simulink model "Copy_of_BatteryPack"  (R2023b)
settings: Solver=VariableStepAuto  StartTime=0.0  StopTime=10.0  RelTol=1e-3
InitFcn:
  | eta=0.992943452611046;
  | Q=5.134436834270520;
  | Qinv=1/Q;
  | Qinv_cells=Qinv+0.01*rand(12,1);
  | delta_t=0.1;
  | delta_t_delta=4;
  | taw=2.410723815561624;
  | R0=0.011163238296886;
  | R0_cells=R0+0.001*rand(12,1);
  | R=0.002515135572506;
  | gamma=61.749752200480295;
  | M0=0.002542395121461;
  | M=0.044341699418566;
  | OCV0=[3.03083668947220,3.16996176507765,3.24654613672245,3.30462471088150,3.35178831826018,3.39207985837564,3.42754280925954,3.45930893308633,3.48845834377828,3.51506471884948,3.53941528250350,3.56229005089512,3.58347680139773,3.60345371361795,3.62204667414497,3.63945293994712,3.65555208129593,3.67025842747189,3.68283722926942,3.69256635796299,3.69934356504319,3.70421492193387,3.70864080668278,3.71251647816700,3.71676450243010,3.72076080442289,3.72459036631361,3.72852113964889,3.73262555664002,3.73679788031633,3.74085805813141,3.74504293170943,3.74937151420852,3.75360503345497,3.75808554938499,3.76253512812700,3.76686713224277,3.77129741354356,3.77568299945893,3.78010899552110,3.78432597237866,3.78866667245794,3.79282973590265,3.79699149175738,3.80102646886227,3.80486901671467,3.80859160652083,3.81234290326678,3.81578374146922,3.81901029060391,3.82246264968075,3.82565270541301,3.82878492908885,3.83182846251259,3.83504605065465,3.83817152994830,3.84120926637331,3.84427045104513,3.84745505461551,3.85048527227548,3.85338258086535,3.85633375142700,3.85903736950342,3.86183294078638,3.86426909473005,3.86668409269911,3.86884960464201,3.87075062579497,3.87260151166861,3.87419873493045,3.87590354579771,3.87742660309802,3.87888623494178,3.88013778482297,3.88172955555187,3.88298517380087,3.88445139467736,3.88588841874555,3.88718906620625,3.88865483707461,3.89034900018679,3.89177308296385,3.89345014882802,3.89492324307466,3.89656804158261,3.89814831273987,3.89970800088682,3.90138268502894,3.90325919869100,3.90466035566401,3.90650715226313,3.90818394205928,3.90991726595604,3.91178869314647,3.91353048350435,3.91535717290223,3.91722943087205,3.91902077537227,3.92094773764149,3.92272669049051,3.92480210727778,3.92665898861166,3.92855163124444,3.93049425931182,3.93233822864100,3.93413808807444,3.93586787406902,3.93781878301823,3.93970352375448,3.94141217835583,3.94337738846496,3.94524781610469,3.94705512196599,3.94889596931986,3.95072813117993,3.95268786149774,3.95437483545637,3.95614043217004,3.95813802002780,3.95988737276266,3.96180145819164,3.96333094922522,3.96513598465409,3.96688905019200,3.96847526303094,3.97032227257873,3.97189764460202,3.97357890138617,3.97507568580842,3.97666308363629,3.97834004990894,3.97972757215233,3.98134719919954,3.98282452838428,3.98434240750033,3.98579080664983,3.98712095624815,3.98848186479248,3.99005169119157,3.99140961007081,3.99272279272243,3.99405266719970,3.99553040552875,3.99686295933407,3.99826042332052,3.99959085613132,4.00118770124588,4.00258756750194,4.00410831223298,4.00564378913664,4.00733579962478,4.00874100440808,4.01049664802522,4.01229894715480,4.01403904622199,4.01578258632489,4.01777261837808,4.01971351876421,4.02181419747090,4.02405411757281,4.02634132187682,4.02844966043338,4.03074821161091,4.03287252710406,4.03519979075052,4.03714724603729,4.03920059502787,4.04119005170582,4.04311251958802,4.04485629277420,4.04687276700581,4.04856655229106,4.05028282064349,4.05188790780758,4.05367115501827,4.05540888556017,4.05715082708000,4.05891707849673,4.06058066558082,4.06255984784218,4.06443355862160,4.06646437679668,4.06828978114252,4.07040446117501,4.07260180541029,4.07472443659757,4.07695226365058,4.07952388568996,4.08211497603818,4.08494517654941,4.08785760361077,4.09108975271414,4.09441257923899,4.09808703497329,4.10213358582538,4.10639223642507,4.11114147862302,4.11656968526475,4.12276605724301,4.13028542232852,4.14480757713318];
  | OCVrel=[-0.000420362949371303,-0.000578339102606499,-0.000548212633161139,-0.000532050376255593,-0.000513855468461292,-0.000495687320522634,-0.000487643250941371,-0.000470920985950642,-0.000461928451583620,-0.000448574992511236,-0.000430345291794665,-0.000415864789930715,-0.000403503275736067,-0.000392608506451838,-0.000381149699535297,-0.000369136346590911,-0.000348156127830507,-0.000324184515919599,-0.000280229092973681,-0.000201932662233446,-0.000110744926726894,-3.79084757376537e-05,7.34820416665105e-08,1.98249344364182e-05,1.89028531032423e-05,1.52778169972465e-05,1.34924868477160e-05,9.23542420261725e-06,-1.46245586440975e-06,-1.45311365618779e-05,-2.47366010229282e-05,-3.53430095058658e-05,-4.35761509840300e-05,-4.95443607046995e-05,-5.59569418266839e-05,-5.71405250985218e-05,-5.58628466608733e-05,-5.23710248925624e-05,-5.22024906444821e-05,-5.10066281299635e-05,-4.60070072284917e-05,-4.39210588487260e-05,-4.17087376582674e-05,-3.79965319780425e-05,-3.52883378328963e-05,-2.96358522826692e-05,-1.93487210265394e-05,-1.76654799578108e-05,-1.10481636980021e-05,-6.29033346947879e-06,-6.43729682754031e-06,-8.99082338466702e-06,-5.97476480532998e-06,-4.62198779734926e-06,-8.45626888598137e-06,-3.55310580626464e-06,1.21105779784145e-06,3.23270957394308e-06,4.65975925632772e-06,6.06047576788568e-06,1.06741421249725e-05,1.27740668978125e-05,1.58322240631086e-05,1.58226143080902e-05,1.77356396535024e-05,1.67297263145319e-05,2.20422014608934e-05,3.24455524629346e-05,4.53671310943400e-05,6.36631547519500e-05,7.65783816690908e-05,9.78737779086299e-05,0.000118072210378981,0.000145052733908454,0.000159053964033644,0.000178615115542580,0.000192951944721033,0.000203745870809340,0.000215887472157157,0.000217389449254637,0.000214080259255523,0.000217368801393146,0.000210680488604522,0.000216791472310507,0.000210807141665482,0.000206892775031066,0.000209889448971827,0.000206480366569060,0.000197477832361696,0.000201878205171392,0.000195991461516702,0.000193299624131949,0.000189225295900371,0.000183015755985024,0.000181030375137689,0.000179058026812520,0.000172630244233569,0.000169739554492468,0.000168470860940041,0.000165673583835095,0.000158761613569570,0.000158310548246597,0.000160768730786868,0.000159274891317150,0.000163654237071923,0.000165646854650985,0.000171009006229332,0.000172960872040281,0.000174059186593325,0.000184792008315373,0.000185457536514424,0.000188497928404933,0.000193540560057086,0.000201967121634793,0.000208651810099923,0.000210203310502306,0.000221327742354831,0.000226934798568295,0.000229022527795167,0.000235980838038274,0.000237393722897026,0.000251416377586933,0.000255669183930939,0.000259582507624291,0.000271756110286130,0.000271428141354407,0.000280338423121521,0.000282159563486788,0.000293698306662556,0.000294690382734668,0.000296368480075595,0.000305852381154249,0.000305547730725772,0.000310124564075650,0.000308910141248888,0.000310910207998593,0.000317136879477080,0.000319966110029179,0.000317781933009713,0.000319714895363342,0.000323633211007860,0.000324670146330631,0.000321258389806546,0.000325090635960723,0.000325756317802870,0.000329299487485483,0.000323022114762843,0.000329687741218402,0.000331335077114761,0.000334366863810491,0.000334190313302610,0.000348244516476559,0.000353619969496185,0.000370645612717080,0.000387424759796793,0.000412712601107454,0.000432980002313212,0.000458081645703528,0.000475316126710853,0.000488710969037302,0.000490229811285922,0.000496997034255361,0.000490732502998424,0.000485413024014050,0.000470031399074122,0.000464225038785084,0.000453594366571016,0.000442947689735187,0.000432361194051228,0.000426870028472560,0.000412534978795853,0.000404144406879032,0.000399500637103100,0.000395361789641937,0.000391903989806764,0.000388094198725783,0.000384493593513828,0.000380890719331740,0.000381944387481867,0.000375725748044827,0.000377689116895975,0.000371263292977880,0.000375401761542324,0.000371961214504098,0.000372140497419301,0.000376623010739057,0.000379713082469440,0.000373305112977953,0.000376271071938692,0.000374048457576144,0.000373866132643822,0.000368451986163444,0.000366513632840686,0.000361449855405437,0.000355758001511034,0.000351852945592445,0.000340424192937049,0.000323803410913197,0.000299570003101876,0.000255297108741397,9.12380218506306e-05];
  | soc_values=[0,0.00500000000000000,0.0100000000000000,0.0150000000000000,0.0200000000000000,0.0250000000000000,0.0300000000000000,0.0350000000000000,0.0400000000000000,0.0450000000000000,0.0500000000000000,0.0550000000000000,0.0600000000000000,0.0650000000000000,0.0700000000000000,0.0750000000000000,0.0800000000000000,0.0850000000000000,0.0900000000000000,0.0950000000000000,0.100000000000000,0.105000000000000,0.110000000000000,0.115000000000000,0.120000000000000,0.125000000000000,0.130000000000000,0.135000000000000,0.140000000000000,0.145000000000000,0.150000000000000,0.155000000000000,0.160000000000000,0.165000000000000,0.170000000000000,0.175000000000000,0.180000000000000,0.185000000000000,0.190000000000000,0.195000000000000,0.200000000000000,0.205000000000000,0.210000000000000,0.215000000000000,0.220000000000000,0.225000000000000,0.230000000000000,0.235000000000000,0.240000000000000,0.245000000000000,0.250000000000000,0.255000000000000,0.260000000000000,0.265000000000000,0.270000000000000,0.275000000000000,0.280000000000000,0.285000000000000,0.290000000000000,0.295000000000000,0.300000000000000,0.305000000000000,0.310000000000000,0.315000000000000,0.320000000000000,0.325000000000000,0.330000000000000,0.335000000000000,0.340000000000000,0.345000000000000,0.350000000000000,0.355000000000000,0.360000000000000,0.365000000000000,0.370000000000000,0.375000000000000,0.380000000000000,0.385000000000000,0.390000000000000,0.395000000000000,0.400000000000000,0.405000000000000,0.410000000000000,0.415000000000000,0.420000000000000,0.425000000000000,0.430000000000000,0.435000000000000,0.440000000000000,0.445000000000000,0.450000000000000,0.455000000000000,0.460000000000000,0.465000000000000,0.470000000000000,0.475000000000000,0.480000000000000,0.485000000000000,0.490000000000000,0.495000000000000,0.500000000000000,0.505000000000000,0.510000000000000,0.515000000000000,0.520000000000000,0.525000000000000,0.530000000000000,0.535000000000000,0.540000000000000,0.545000000000000,0.550000000000000,0.555000000000000,0.560000000000000,0.565000000000000,0.570000000000000,0.575000000000000,0.580000000000000,0.585000000000000,0.590000000000000,0.595000000000000,0.600000000000000,0.605000000000000,0.610000000000000,0.615000000000000,0.620000000000000,0.625000000000000,0.630000000000000,0.635000000000000,0.640000000000000,0.645000000000000,0.650000000000000,0.655000000000000,0.660000000000000,0.665000000000000,0.670000000000000,0.675000000000000,0.680000000000000,0.685000000000000,0.690000000000000,0.695000000000000,0.700000000000000,0.705000000000000,0.710000000000000,0.715000000000000,0.720000000000000,0.725000000000000,0.730000000000000,0.735000000000000,0.740000000000000,0.745000000000000,0.750000000000000,0.755000000000000,0.760000000000000,0.765000000000000,0.770000000000000,0.775000000000000,0.780000000000000,0.785000000000000,0.790000000000000,0.795000000000000,0.800000000000000,0.805000000000000,0.810000000000000,0.815000000000000,0.820000000000000,0.825000000000000,0.830000000000000,0.835000000000000,0.840000000000000,0.845000000000000,0.850000000000000,0.855000000000000,0.860000000000000,0.865000000000000,0.870000000000000,0.875000000000000,0.880000000000000,0.885000000000000,0.890000000000000,0.895000000000000,0.900000000000000,0.905000000000000,0.910000000000000,0.915000000000000,0.920000000000000,0.925000000000000,0.930000000000000,0.935000000000000,0.940000000000000,0.945000000000000,0.950000000000000,0.955000000000000,0.960000000000000,0.965000000000000,0.970000000000000,0.975000000000000,0.980000000000000,0.985000000000000,0.990000000000000,0.995000000000000,1];
  | OCV_values=OCV0+25*OCVrel;
  | dZ = soc_values(2) - soc_values(1); % Find spacing of SOC vector
  | dUdZ = diff(OCV_values)/dZ; % Scaled forward finite difference
  | dOCV = ([dUdZ(1) dUdZ] + [dUdZ dUdZ(end)])/2; % Avg of fwd/bkwd diffs
  | SigmaX0 = diag([1e-3 1e-3 1e-2]); % uncertainty of initial state
  | sigmaV = 2e-1; % uncertainty of voltage sensor, output equation
  | sigmaW = 1e1; % uncertainty of current sensor, state equation
  | vbar=0;
  | w_bar=0;
  | nR=0.004;
  | nQ=0.05;
  | ek=0.01;
  | Vmax=4.2;
  | Vmin=2.7;
  | Imax=2*Q;
  | Standby=0;
  | Charging=1;
  | Discharging=2;
  | load('BattCrntDrvCycle.mat');
undefined symbols (not defined in the file): AUX0_OV, AUX1_OV, AUX2_OV, AUX3_OV, AUX4_OV, CELL_OV, CELL_UV, CellVoltages, Fault, FAULT_SUM, NCHAN, PackCurrentChg, PackCurrentDis, PackVoltage, Temperature
libraries: fl_lib x38, nesl_utility x25, simulink x15, ee_lib x8, eeGeneralControl x7, batt_lib x7, hdlsllib x3
(part 2 of 3)

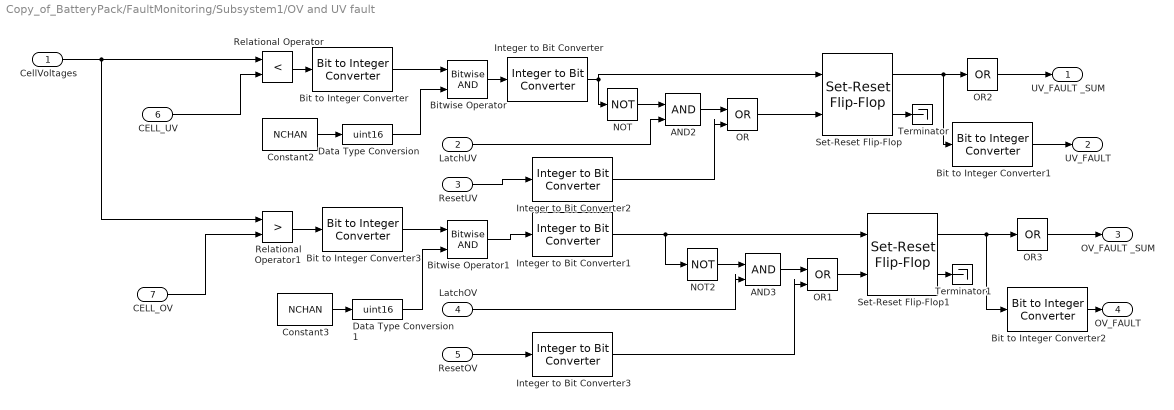
== system Copy_of_BatteryPack/FaultMonitoring/Subsystem1/OV and UV fault ==
  CellVoltages : Inport
  LatchUV : Inport  Port=2
  ResetUV : Inport  Port=3
  LatchOV : Inport  Port=4
  ResetOV : Inport  Port=5
  CELL_UV : Inport  Port=6
  CELL_OV : Inport  Port=7
  AND2 : Logic  IconShape=distinctive  AllPortsSameDT=off  OutDataTypeStr=boolean
  AND3 : Logic  IconShape=distinctive  AllPortsSameDT=off  OutDataTypeStr=boolean
  Bit to Integer Converter{,1..3} (4 alike) : simulink/Logic and Bit Operations/Bit to Integer Converter  nbits=16  bitOrder=MSB first  signedOutputValues=Unsigned  outDtype=Inherit via internal rule  outDtypeSigned=Inherit via internal rule
  Bitwise Operator : simulink/Logic and Bit Operations/Bitwise Operator  logicop=AND  UseBitMask=off  NumInputPorts=2  BitMask=bin2dec('11011001')  BitMaskRealWorld=Stored Integer
  Bitwise Operator1 : simulink/Logic and Bit Operations/Bitwise Operator  logicop=AND  UseBitMask=off  NumInputPorts=2  BitMask=bin2dec('11011001')  BitMaskRealWorld=Stored Integer
  Constant2 : Constant  Value=NCHAN
  Constant3 : Constant  Value=NCHAN
  Data Type Conversion : DataTypeConversion  OutDataTypeStr=uint16  SaturateOnIntegerOverflow=off  RndMeth=Floor
  Data Type Conversion1 : DataTypeConversion  OutDataTypeStr=uint16  SaturateOnIntegerOverflow=off  RndMeth=Floor
  Integer to Bit Converter{,1..3} (4 alike) : simulink/Logic and Bit Operations/Integer to Bit Converter  nbits=16  signedInputValues=Unsigned  bitOrder=MSB first  outDtype=Inherit via internal rule
  NOT : Logic  Operator=NOT  IconShape=distinctive  AllPortsSameDT=off  OutDataTypeStr=boolean
  NOT2 : Logic  Operator=NOT  IconShape=distinctive  AllPortsSameDT=off  OutDataTypeStr=boolean
  OR : Logic  Operator=OR  IconShape=distinctive  AllPortsSameDT=off  OutDataTypeStr=boolean
  OR1 : Logic  Operator=OR  IconShape=distinctive  AllPortsSameDT=off  OutDataTypeStr=boolean
  OR2 : Logic  Operator=OR  Inputs=1  IconShape=distinctive  AllPortsSameDT=off  OutDataTypeStr=boolean
  OR3 : Logic  Operator=OR  Inputs=1  IconShape=distinctive  AllPortsSameDT=off  OutDataTypeStr=boolean
  Relational Operator : RelationalOperator  Operator=<  OutDataTypeStr=boolean  RndMeth=Simplest  InputSameDT=off
  Relational Operator1 : RelationalOperator  Operator=>  OutDataTypeStr=boolean  RndMeth=Simplest  InputSameDT=off
  Set-Reset Flip-Flop : eeGeneralControl/Set-Reset Flip-Flop  LabelModeActiveChoice=Discrete  UndefState=Set  Q0=0  Ts=-1
      settings: LibrarySourceBlock=ee_sl_lib/General Control/Set-Reset Flip-Flop
  Set-Reset Flip-Flop1 : eeGeneralControl/Set-Reset Flip-Flop  LabelModeActiveChoice=Discrete  UndefState=Set  Q0=0  Ts=-1
      settings: LibrarySourceBlock=ee_sl_lib/General Control/Set-Reset Flip-Flop
  Terminator : Terminator
  Terminator1 : Terminator
  UV_FAULT _SUM : Outport
  UV_FAULT : Outport  Port=2
  OV_FAULT _SUM : Outport  Port=3
  OV_FAULT : Outport  Port=4
  wires:
  CellVoltages/1 -> Relational Operator1/1, Relational Operator/1
  CELL_UV/1 -> Relational Operator/2
  CELL_OV/1 -> Relational Operator1/2
  Relational Operator/1 -> Bit to Integer Converter/1
  Constant2/1 -> Data Type Conversion/1
  Relational Operator1/1 -> Bit to Integer Converter3/1
  Constant3/1 -> Data Type Conversion1/1
  Bitwise Operator/1 -> Integer to Bit Converter/1
  NOT/1 -> AND2/1
  LatchUV/1 -> AND2/2
  AND2/1 -> OR/1
  ResetUV/1 -> Integer to Bit Converter2/1
  OR/1 -> Set-Reset Flip-Flop/2
  Set-Reset Flip-Flop/1 -> Bit to Integer Converter1/1, OR2/1
  AND3/1 -> OR1/1
  ResetOV/1 -> Integer to Bit Converter3/1
  LatchOV/1 -> AND3/2
  NOT2/1 -> AND3/1
  OR1/1 -> Set-Reset Flip-Flop1/2
  Bitwise Operator1/1 -> Integer to Bit Converter1/1
  Set-Reset Flip-Flop/2 -> Terminator/1
  Set-Reset Flip-Flop1/2 -> Terminator1/1
  Set-Reset Flip-Flop1/1 -> Bit to Integer Converter2/1, OR3/1
  OR2/1 -> UV_FAULT _SUM/1
  OR3/1 -> OV_FAULT _SUM/1
  Bit to Integer Converter/1 -> Bitwise Operator/1
  Data Type Conversion/1 -> Bitwise Operator/2
  Integer to Bit Converter/1 -> Set-Reset Flip-Flop/1, NOT/1
  Bit to Integer Converter1/1 -> UV_FAULT/1
  Bit to Integer Converter2/1 -> OV_FAULT/1
  Integer to Bit Converter1/1 -> Set-Reset Flip-Flop1/1, NOT2/1
  Bit to Integer Converter3/1 -> Bitwise Operator1/1
  Data Type Conversion1/1 -> Bitwise Operator1/2
  Integer to Bit Converter2/1 -> OR/2
  Integer to Bit Converter3/1 -> OR1/2

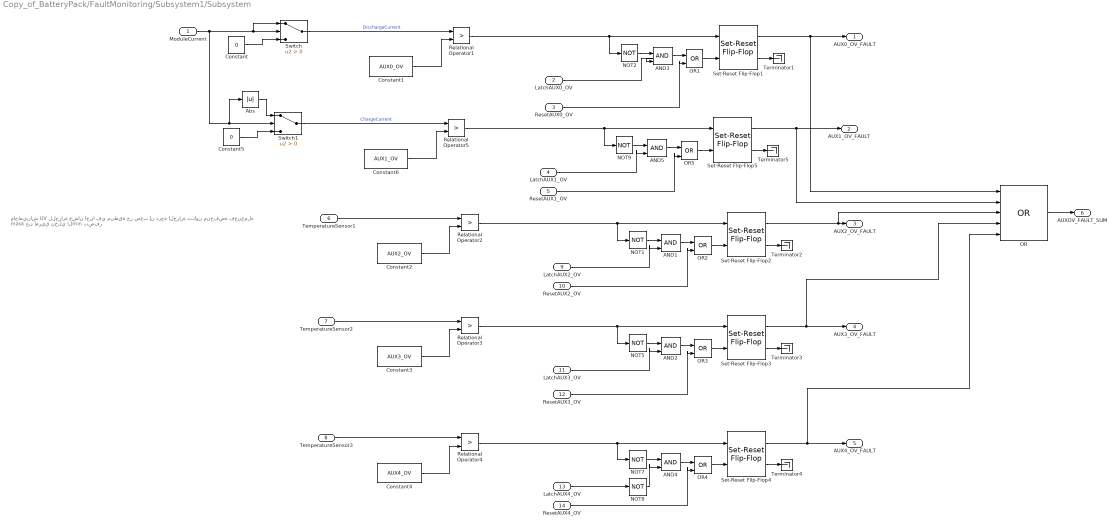
== system Copy_of_BatteryPack/FaultMonitoring/Subsystem1/Subsystem ==
  note: ماحطيناش UV للحرارة عشان احنا في منطقة حر صعب إن درجة الحرارة تكون منخفضة
      | فعنعمله mask عن طريق نخلي الmin بصفر
  ModuleCurrent : Inport
  LatchAUX0_OV : Inport  Port=2
  ResetAUX0_OV : Inport  Port=3
  LatchAUX1_OV : Inport  Port=4
  ResetAUX1_OV : Inport  Port=5
  TemperatureSensor1 : Inport  Port=6
  TemperatureSensor2 : Inport  Port=7
  TemperatureSensor3 : Inport  Port=8
  LatchAUX2_OV : Inport  Port=9
  ResetAUX2_OV : Inport  Port=10
  LatchAUX3_OV : Inport  Port=11
  ResetAUX3_OV : Inport  Port=12
  LatchAUX4_OV : Inport  Port=13
  ResetAUX4_OV : Inport  Port=14
  AND{1..5} (5 alike) : Logic  IconShape=distinctive  AllPortsSameDT=off  OutDataTypeStr=boolean
  Abs : Abs  SaturateOnIntegerOverflow=off
  Constant : Constant  Value=0
  Constant1 : Constant  Value=AUX0_OV
  Constant2 : Constant  Value=AUX2_OV
  Constant3 : Constant  Value=AUX3_OV
  Constant4 : Constant  Value=AUX4_OV
  Constant5 : Constant  Value=0
  Constant6 : Constant  Value=AUX1_OV
  NOT{1..2,5,7..9} (6 alike) : Logic  Operator=NOT  IconShape=distinctive  AllPortsSameDT=off  OutDataTypeStr=boolean
  OR : Logic  Operator=OR  Inputs=5  AllPortsSameDT=off  OutDataTypeStr=boolean
  OR{1..5} (5 alike) : Logic  Operator=OR  IconShape=distinctive  AllPortsSameDT=off  OutDataTypeStr=boolean
  Relational Operator{1..5} (5 alike) : RelationalOperator  Operator=>  OutDataTypeStr=boolean  RndMeth=Simplest  InputSameDT=off
  Set-Reset Flip-Flop{1..5} (5 alike) : eeGeneralControl/Set-Reset Flip-Flop  LabelModeActiveChoice=Discrete  UndefState=Set  Q0=0  Ts=-1
      settings: LibrarySourceBlock=ee_sl_lib/General Control/Set-Reset Flip-Flop
  Switch : Switch  Criteria=u2 > Threshold  SaturateOnIntegerOverflow=off  InputSameDT=off
  Switch1 : Switch  Criteria=u2 > Threshold  SaturateOnIntegerOverflow=off  InputSameDT=off
  Terminator{1..5} (5 alike) : Terminator
  AUX0_OV_FAULT : Outport
  AUX1_OV_FAULT : Outport  Port=2
  AUX2_OV_FAULT : Outport  Port=3
  AUX3_OV_FAULT : Outport  Port=4
  AUX4_OV_FAULT : Outport  Port=5
  AUXOV_FAULT_SUM : Outport  Port=6
  wires:
  ResetAUX0_OV/1 -> OR1/2
  NOT2/1 -> AND3/1
  LatchAUX0_OV/1 -> AND3/2
  AND3/1 -> OR1/1
  Constant1/1 -> Relational Operator1/2
  Set-Reset Flip-Flop1/1 -> OR/1, AUX0_OV_FAULT/1
  Set-Reset Flip-Flop1/2 -> Terminator1/1
  OR1/1 -> Set-Reset Flip-Flop1/2
  Relational Operator1/1 -> NOT2/1, Set-Reset Flip-Flop1/1
  ResetAUX2_OV/1 -> OR2/2
  OR2/1 -> Set-Reset Flip-Flop2/2
  Set-Reset Flip-Flop2/2 -> Terminator2/1
  Constant2/1 -> Relational Operator2/2
  LatchAUX2_OV/1 -> AND1/2
  AND1/1 -> OR2/1
  Relational Operator2/1 -> NOT1/1, Set-Reset Flip-Flop2/1
  Set-Reset Flip-Flop2/1 -> OR/3, AUX2_OV_FAULT/1
  NOT1/1 -> AND1/1
  TemperatureSensor1/1 -> Relational Operator2/1
  TemperatureSensor2/1 -> Relational Operator3/1
  Relational Operator3/1 -> NOT5/1, Set-Reset Flip-Flop3/1
  AND2/1 -> OR3/1
  Constant3/1 -> Relational Operator3/2
  Set-Reset Flip-Flop3/2 -> Terminator3/1
  ResetAUX3_OV/1 -> OR3/2
  OR3/1 -> Set-Reset Flip-Flop3/2
  Set-Reset Flip-Flop3/1 -> OR/4, AUX3_OV_FAULT/1
  NOT5/1 -> AND2/1
  LatchAUX3_OV/1 -> AND2/2
  TemperatureSensor3/1 -> Relational Operator4/1
  Relational Operator4/1 -> NOT7/1, Set-Reset Flip-Flop4/1
  AND4/1 -> OR4/1
  Constant4/1 -> Relational Operator4/2
  Set-Reset Flip-Flop4/2 -> Terminator4/1
  ResetAUX4_OV/1 -> OR4/2
  OR4/1 -> Set-Reset Flip-Flop4/2
  LatchAUX4_OV/1 -> NOT8/1
  NOT7/1 -> AND4/1
  NOT8/1 -> AND4/2
  Set-Reset Flip-Flop4/1 -> OR/5, AUX4_OV_FAULT/1
  OR/1 -> AUXOV_FAULT_SUM/1
  Constant/1 -> Switch/3
  Switch/1 -> Relational Operator1/1  "DischargeCurrent"
  ResetAUX1_OV/1 -> OR5/2
  OR5/1 -> Set-Reset Flip-Flop5/2
  Set-Reset Flip-Flop5/2 -> Terminator5/1
  Constant6/1 -> Relational Operator5/2
  AND5/1 -> OR5/1
  Switch1/1 -> Relational Operator5/1  "ChargeCurrent"
  Relational Operator5/1 -> NOT9/1, Set-Reset Flip-Flop5/1
  Set-Reset Flip-Flop5/1 -> OR/2, AUX1_OV_FAULT/1
  NOT9/1 -> AND5/1
  LatchAUX1_OV/1 -> AND5/2
  ModuleCurrent/1 -> Switch/1, Switch/2, Switch1/2, Abs/1
  Constant5/1 -> Switch1/3
  Abs/1 -> Switch1/1

== system Copy_of_BatteryPack/Subsystem3/Battery pack3/Subsystem10 ==
  Balance Command : Inport
  Diode : ee_lib/Semiconductors & Converters/Diode  ModelType=ee.enum.diode.modelType.pwl  TableType=ee.enum.diode.tableType.IfMat  IfMat=[.07, .12, .19, 1.75, 4.24, 7.32, 11.2; .16, .3, .72, 2.14, 5.02, 8.35, 13.12] A  VfMat=[.9, 1.15, 1.25, 1.5, 1.75, 2.17, 2.6, 2.85; .58, .68, .75, 1.1, 1.38, 1.77, 2.27, 2.7] V  TjVec=[25, 125] degC  VfVec=[.5, .7, .9, 1.3, 1.7, 2.1, 2.5] V  IfVec=[.1, .2, .5, 1, 2, 4, 7, 10] A  Vf=0.6 V  Ron=0.3 Ohm  Goff=1e-8 S  prmExp=ee.enum.diode.expParam.useTwo  I12=[.0137, .545] A  V12=[.6, .7] V  RS=0 Ohm  Tmeas=25 degC  IS=1e-12 A  ec=1  I1=0.0137 A  V1=0.6 V  N_series=1  N_parallel=1  ZenerEnable=false  Rz=0.3 Ohm  BV=inf V  C_param=ee.enum.diode.capParam.fixed  CJ=0 pF  CJ0=5 pF  Vvec=[.1, 10, 100] V  Cvec=[3.5, 1, .4] pF  VJ=1 V  Mgrad=0.5  FC=0.5  Q_param=ee.enum.diode.recoveryParam.off  iRM=-7.15 A  iF=4 A  didt=-750 A/us  trr_factor=3  trr=115 ns  Qrr=150 nA*s  Vr=-600 V  Ls=150 nH  Erec=0.03 J  TT=50 ns  tau=100 ns  T_param=ee.enum.diode.temperatureParam.off  Tdevice=25 degC  I1_T2=0.245 A  V1_T2=0.5 V  IS_T2=1.25e-7 A  Tmeas2=125 degC  XTI_param=ee.enum.diode.xtiParam.pn  XTI=3  EG_param=ee.enum.diode.egapParam.material_si  EG=1.11 eV  dBVdT=0 V/K  enable_faults=simscape.enum.onoff.off  fault_action=simscape.enum.assert.action.none  fault_types=ee.enum.diode.faults.open  tau_fault=1e-3 s  IfMat_faulted=[.07, .12, .19, 1.75, 4.24, 7.32, 11.2; .16, .3, .72, 2.14, 4.02, 6.35, 9.12] A  VfMat_faulted=[.9, 1.15, 1.25, 1.5, 1.75, 2.17, 2.6, 2.85; .58, .68, .75, 1.1, 1.38, 1.77, 2.27, 2.7] V  VfVec_faulted=[.5, .7, .9, 1.3, 1.7, 2.1, 2.5] V  IfVec_faulted=[.1, .2, .5, 1, 2, 4, 7, 10] A  Ropen_faulted=1000 Ohm  Gshort_faulted=1000 1/Ohm  Vf_faulted=0.6 V  Ron_faulted=0.3 Ohm  Goff_faulted=1e-8 S  I12_faulted=[.0137, .545] A  V12_faulted=[.6, .7] V  IS_faulted=1e-12 A  ec_faulted=1  I1_faulted=0.0137 A  V1_faulted=0.6 V  RS_faulted=0 Ohm  Rz_faulted=0.3 Ohm  BV_faulted=inf V  Cscale_faulted=100  fault_trigger=ee.enum.faults.faultTrigger.temporal  t_fault=inf s  max_permissible_voltage=inf V  n_fail_on_voltage=1  max_permissible_current=inf A  t_fail_on_current=1 s  max_permissible_dVdt=inf V/s  enable_fault_input=simscape.enum.onoff.off  i_specify=off  i_priority=None  i=0 A  i_nominal_specify=off  i_nominal_unit=A  i_nominal_value=1  v_specify=off  v_priority=None  v=0 V  v_nominal_specify=off  v_nominal_unit=V  v_nominal_value=1  v_capacitor_specify=off  v_capacitor_priority=None  v_capacitor=0 V  v_capacitor_nominal_specify=off  v_capacitor_nominal_unit=V  v_capacitor_nominal_value=1  faulted_specify=off  faulted_priority=None  faulted=0  faulted_nominal_specify=off  faulted_nominal_unit=1  faulted_nominal_value=1  i_diode_specify=off  i_diode_priority=None  i_diode=0 A  i_diode_nominal_specify=off  i_diode_nominal_unit=A  i_diode_nominal_value=1  v_diode_specify=off  v_diode_priority=None  v_diode=0 V  v_diode_nominal_specify=off  v_diode_nominal_unit=V  v_diode_nominal_value=1  i_capacitor_specify=off  i_capacitor_priority=None  i_capacitor=0 A  i_capacitor_nominal_specify=off  i_capacitor_nominal_unit=A  i_capacitor_nominal_value=1  power_dissipated_specify=off  power_dissipated_priority=None  power_dissipated=0 W  power_dissipated_nominal_specify=off  power_dissipated_nominal_unit=W  power_dissipated_nominal_value=1  fidelity_level=ee.enum.diode.fidelity.includeChargeDyn  rec_loss_model=ee.enum.diode.reverseRecoveryModel.fixed  ErecVal=0 J  scaleWithIandV=true  ErecMat=zeros(2, 3) J  TjrecVec=[298.15, 398.15] K  IfrecVec=[.1, 1, 10] A  IrecVal=10 A  VrecVal=10 V  tFilter=1 / 1000 / 100 s  max_permissible_temperature=inf K  t_fail_on_temperature=1 s  thermal_network_parameterization=ee.enum.thermalNetworkTopology.junctionCase  Rth=[0, 10] K/W  Rth_Cauer=[1, 3, 10] K/W  Rth_Foster=[4, 6] K/W  thermal_mass_parameterization=ee.enum.thermalNetwork.timeconstant  thermal_mass=[0, 1] J/K  thermal_mass_Cauer=[.1, .3, 1] J/K  thermal_mass_Foster=[1.5, 3] J/K  thermal_time_constant=[0, 10] s  thermal_time_constant_Cauer=[1, 3, 10] s  thermal_time_constant_Foster=[6, 18] s  thermal_mass_initial_temperatures=[25, 25] degC  thermal_mass_initial_temperatures_Cauer=[25, 25, 25] degC  junction_thermal_mass=0.01 J/K  Tvec_initial_Foster=[25, 25, 25, 25] degC  no_thermal_network=0  junction_temperature_specify=off  junction_temperature_priority=None  junction_temperature=25 degC  junction_temperature_nominal_specify=off  junction_temperature_nominal_unit=degC  junction_temperature_nominal_value=1
  Resistor : fl_lib/Electrical/Electrical Elements/Resistor  R=33 Ohm  i_specify=off  i_priority=None  i=0 A  i_nominal_specify=off  i_nominal_unit=A  i_nominal_value=1  v_specify=off  v_priority=None  v=0 V  v_nominal_specify=off  v_nominal_unit=V  v_nominal_value=1
  Simulink-PS Converter : nesl_utility/Simulink-PS Converter  PhysicalDomain=network_engine_domain  SubClassName=ps_input  LeftPortType=input  RightPortType=output  PseudoPeriodic=off  Frequencies=[]  NoiseDistribution=none  NoiseParameters=[]  Unit=1  AffineConversion=off  FilteringAndDerivatives=provide  SimscapeFilterOrder=1  InputFilterTimeConstant=0.001  UdotUserProvided=0
  Switch : fl_lib/Electrical/Electrical Elements/Switch  R_closed=0.01 Ohm  G_open=1e-8 1/Ohm  Threshold=0.5  i_specify=off  i_priority=None  i=0 A  i_nominal_specify=off  i_nominal_unit=A  i_nominal_value=1  v_specify=off  v_priority=None  v=0 V  v_nominal_specify=off  v_nominal_unit=V  v_nominal_value=1
  +ve : PMIOPort  Side=Right
  -ve : PMIOPort  Port=2  Side=Right
  wires:
  Balance Command/1 -> Simulink-PS Converter/1
  connections:
  Diode/RConn1 -- Switch/LConn1
  Resistor/RConn1 -- Diode/LConn1
  Resistor/LConn1 -- +ve/RConn1
  -ve/RConn1 -- Switch/RConn2
  Simulink-PS Converter/RConn1 -- Switch/RConn1

== system Copy_of_BatteryPack/Subsystem3/Battery pack3/Subsystem11 ==
  Balance Command : Inport
  Diode : ee_lib/Semiconductors & Converters/Diode  ModelType=ee.enum.diode.modelType.pwl  TableType=ee.enum.diode.tableType.IfMat  IfMat=[.07, .12, .19, 1.75, 4.24, 7.32, 11.2; .16, .3, .72, 2.14, 5.02, 8.35, 13.12] A  VfMat=[.9, 1.15, 1.25, 1.5, 1.75, 2.17, 2.6, 2.85; .58, .68, .75, 1.1, 1.38, 1.77, 2.27, 2.7] V  TjVec=[25, 125] degC  VfVec=[.5, .7, .9, 1.3, 1.7, 2.1, 2.5] V  IfVec=[.1, .2, .5, 1, 2, 4, 7, 10] A  Vf=0.6 V  Ron=0.3 Ohm  Goff=1e-8 S  prmExp=ee.enum.diode.expParam.useTwo  I12=[.0137, .545] A  V12=[.6, .7] V  RS=0 Ohm  Tmeas=25 degC  IS=1e-12 A  ec=1  I1=0.0137 A  V1=0.6 V  N_series=1  N_parallel=1  ZenerEnable=false  Rz=0.3 Ohm  BV=inf V  C_param=ee.enum.diode.capParam.fixed  CJ=0 pF  CJ0=5 pF  Vvec=[.1, 10, 100] V  Cvec=[3.5, 1, .4] pF  VJ=1 V  Mgrad=0.5  FC=0.5  Q_param=ee.enum.diode.recoveryParam.off  iRM=-7.15 A  iF=4 A  didt=-750 A/us  trr_factor=3  trr=115 ns  Qrr=150 nA*s  Vr=-600 V  Ls=150 nH  Erec=0.03 J  TT=50 ns  tau=100 ns  T_param=ee.enum.diode.temperatureParam.off  Tdevice=25 degC  I1_T2=0.245 A  V1_T2=0.5 V  IS_T2=1.25e-7 A  Tmeas2=125 degC  XTI_param=ee.enum.diode.xtiParam.pn  XTI=3  EG_param=ee.enum.diode.egapParam.material_si  EG=1.11 eV  dBVdT=0 V/K  enable_faults=simscape.enum.onoff.off  fault_action=simscape.enum.assert.action.none  fault_types=ee.enum.diode.faults.open  tau_fault=1e-3 s  IfMat_faulted=[.07, .12, .19, 1.75, 4.24, 7.32, 11.2; .16, .3, .72, 2.14, 4.02, 6.35, 9.12] A  VfMat_faulted=[.9, 1.15, 1.25, 1.5, 1.75, 2.17, 2.6, 2.85; .58, .68, .75, 1.1, 1.38, 1.77, 2.27, 2.7] V  VfVec_faulted=[.5, .7, .9, 1.3, 1.7, 2.1, 2.5] V  IfVec_faulted=[.1, .2, .5, 1, 2, 4, 7, 10] A  Ropen_faulted=1000 Ohm  Gshort_faulted=1000 1/Ohm  Vf_faulted=0.6 V  Ron_faulted=0.3 Ohm  Goff_faulted=1e-8 S  I12_faulted=[.0137, .545] A  V12_faulted=[.6, .7] V  IS_faulted=1e-12 A  ec_faulted=1  I1_faulted=0.0137 A  V1_faulted=0.6 V  RS_faulted=0 Ohm  Rz_faulted=0.3 Ohm  BV_faulted=inf V  Cscale_faulted=100  fault_trigger=ee.enum.faults.faultTrigger.temporal  t_fault=inf s  max_permissible_voltage=inf V  n_fail_on_voltage=1  max_permissible_current=inf A  t_fail_on_current=1 s  max_permissible_dVdt=inf V/s  enable_fault_input=simscape.enum.onoff.off  i_specify=off  i_priority=None  i=0 A  i_nominal_specify=off  i_nominal_unit=A  i_nominal_value=1  v_specify=off  v_priority=None  v=0 V  v_nominal_specify=off  v_nominal_unit=V  v_nominal_value=1  v_capacitor_specify=off  v_capacitor_priority=None  v_capacitor=0 V  v_capacitor_nominal_specify=off  v_capacitor_nominal_unit=V  v_capacitor_nominal_value=1  faulted_specify=off  faulted_priority=None  faulted=0  faulted_nominal_specify=off  faulted_nominal_unit=1  faulted_nominal_value=1  i_diode_specify=off  i_diode_priority=None  i_diode=0 A  i_diode_nominal_specify=off  i_diode_nominal_unit=A  i_diode_nominal_value=1  v_diode_specify=off  v_diode_priority=None  v_diode=0 V  v_diode_nominal_specify=off  v_diode_nominal_unit=V  v_diode_nominal_value=1  i_capacitor_specify=off  i_capacitor_priority=None  i_capacitor=0 A  i_capacitor_nominal_specify=off  i_capacitor_nominal_unit=A  i_capacitor_nominal_value=1  power_dissipated_specify=off  power_dissipated_priority=None  power_dissipated=0 W  power_dissipated_nominal_specify=off  power_dissipated_nominal_unit=W  power_dissipated_nominal_value=1  fidelity_level=ee.enum.diode.fidelity.includeChargeDyn  rec_loss_model=ee.enum.diode.reverseRecoveryModel.fixed  ErecVal=0 J  scaleWithIandV=true  ErecMat=zeros(2, 3) J  TjrecVec=[298.15, 398.15] K  IfrecVec=[.1, 1, 10] A  IrecVal=10 A  VrecVal=10 V  tFilter=1 / 1000 / 100 s  max_permissible_temperature=inf K  t_fail_on_temperature=1 s  thermal_network_parameterization=ee.enum.thermalNetworkTopology.junctionCase  Rth=[0, 10] K/W  Rth_Cauer=[1, 3, 10] K/W  Rth_Foster=[4, 6] K/W  thermal_mass_parameterization=ee.enum.thermalNetwork.timeconstant  thermal_mass=[0, 1] J/K  thermal_mass_Cauer=[.1, .3, 1] J/K  thermal_mass_Foster=[1.5, 3] J/K  thermal_time_constant=[0, 10] s  thermal_time_constant_Cauer=[1, 3, 10] s  thermal_time_constant_Foster=[6, 18] s  thermal_mass_initial_temperatures=[25, 25] degC  thermal_mass_initial_temperatures_Cauer=[25, 25, 25] degC  junction_thermal_mass=0.01 J/K  Tvec_initial_Foster=[25, 25, 25, 25] degC  no_thermal_network=0  junction_temperature_specify=off  junction_temperature_priority=None  junction_temperature=25 degC  junction_temperature_nominal_specify=off  junction_temperature_nominal_unit=degC  junction_temperature_nominal_value=1
  Resistor : fl_lib/Electrical/Electrical Elements/Resistor  R=33 Ohm  i_specify=off  i_priority=None  i=0 A  i_nominal_specify=off  i_nominal_unit=A  i_nominal_value=1  v_specify=off  v_priority=None  v=0 V  v_nominal_specify=off  v_nominal_unit=V  v_nominal_value=1
  Simulink-PS Converter : nesl_utility/Simulink-PS Converter  PhysicalDomain=network_engine_domain  SubClassName=ps_input  LeftPortType=input  RightPortType=output  PseudoPeriodic=off  Frequencies=[]  NoiseDistribution=none  NoiseParameters=[]  Unit=1  AffineConversion=off  FilteringAndDerivatives=provide  SimscapeFilterOrder=1  InputFilterTimeConstant=0.001  UdotUserProvided=0
  Switch : fl_lib/Electrical/Electrical Elements/Switch  R_closed=0.01 Ohm  G_open=1e-8 1/Ohm  Threshold=0.5  i_specify=off  i_priority=None  i=0 A  i_nominal_specify=off  i_nominal_unit=A  i_nominal_value=1  v_specify=off  v_priority=None  v=0 V  v_nominal_specify=off  v_nominal_unit=V  v_nominal_value=1
  +ve : PMIOPort  Side=Right
  -ve : PMIOPort  Port=2  Side=Right
  wires:
  Balance Command/1 -> Simulink-PS Converter/1
  connections:
  Diode/RConn1 -- Switch/LConn1
  Resistor/RConn1 -- Diode/LConn1
  Resistor/LConn1 -- +ve/RConn1
  -ve/RConn1 -- Switch/RConn2
  Simulink-PS Converter/RConn1 -- Switch/RConn1

== system Copy_of_BatteryPack/Subsystem3/Battery pack3/Subsystem5 ==
  Balance Command : Inport
  Diode : ee_lib/Semiconductors & Converters/Diode  ModelType=ee.enum.diode.modelType.pwl  TableType=ee.enum.diode.tableType.IfMat  IfMat=[.07, .12, .19, 1.75, 4.24, 7.32, 11.2; .16, .3, .72, 2.14, 5.02, 8.35, 13.12] A  VfMat=[.9, 1.15, 1.25, 1.5, 1.75, 2.17, 2.6, 2.85; .58, .68, .75, 1.1, 1.38, 1.77, 2.27, 2.7] V  TjVec=[25, 125] degC  VfVec=[.5, .7, .9, 1.3, 1.7, 2.1, 2.5] V  IfVec=[.1, .2, .5, 1, 2, 4, 7, 10] A  Vf=0.6 V  Ron=0.3 Ohm  Goff=1e-8 S  prmExp=ee.enum.diode.expParam.useTwo  I12=[.0137, .545] A  V12=[.6, .7] V  RS=0 Ohm  Tmeas=25 degC  IS=1e-12 A  ec=1  I1=0.0137 A  V1=0.6 V  N_series=1  N_parallel=1  ZenerEnable=false  Rz=0.3 Ohm  BV=inf V  C_param=ee.enum.diode.capParam.fixed  CJ=0 pF  CJ0=5 pF  Vvec=[.1, 10, 100] V  Cvec=[3.5, 1, .4] pF  VJ=1 V  Mgrad=0.5  FC=0.5  Q_param=ee.enum.diode.recoveryParam.off  iRM=-7.15 A  iF=4 A  didt=-750 A/us  trr_factor=3  trr=115 ns  Qrr=150 nA*s  Vr=-600 V  Ls=150 nH  Erec=0.03 J  TT=50 ns  tau=100 ns  T_param=ee.enum.diode.temperatureParam.off  Tdevice=25 degC  I1_T2=0.245 A  V1_T2=0.5 V  IS_T2=1.25e-7 A  Tmeas2=125 degC  XTI_param=ee.enum.diode.xtiParam.pn  XTI=3  EG_param=ee.enum.diode.egapParam.material_si  EG=1.11 eV  dBVdT=0 V/K  enable_faults=simscape.enum.onoff.off  fault_action=simscape.enum.assert.action.none  fault_types=ee.enum.diode.faults.open  tau_fault=1e-3 s  IfMat_faulted=[.07, .12, .19, 1.75, 4.24, 7.32, 11.2; .16, .3, .72, 2.14, 4.02, 6.35, 9.12] A  VfMat_faulted=[.9, 1.15, 1.25, 1.5, 1.75, 2.17, 2.6, 2.85; .58, .68, .75, 1.1, 1.38, 1.77, 2.27, 2.7] V  VfVec_faulted=[.5, .7, .9, 1.3, 1.7, 2.1, 2.5] V  IfVec_faulted=[.1, .2, .5, 1, 2, 4, 7, 10] A  Ropen_faulted=1000 Ohm  Gshort_faulted=1000 1/Ohm  Vf_faulted=0.6 V  Ron_faulted=0.3 Ohm  Goff_faulted=1e-8 S  I12_faulted=[.0137, .545] A  V12_faulted=[.6, .7] V  IS_faulted=1e-12 A  ec_faulted=1  I1_faulted=0.0137 A  V1_faulted=0.6 V  RS_faulted=0 Ohm  Rz_faulted=0.3 Ohm  BV_faulted=inf V  Cscale_faulted=100  fault_trigger=ee.enum.faults.faultTrigger.temporal  t_fault=inf s  max_permissible_voltage=inf V  n_fail_on_voltage=1  max_permissible_current=inf A  t_fail_on_current=1 s  max_permissible_dVdt=inf V/s  enable_fault_input=simscape.enum.onoff.off  i_specify=off  i_priority=None  i=0 A  i_nominal_specify=off  i_nominal_unit=A  i_nominal_value=1  v_specify=off  v_priority=None  v=0 V  v_nominal_specify=off  v_nominal_unit=V  v_nominal_value=1  v_capacitor_specify=off  v_capacitor_priority=None  v_capacitor=0 V  v_capacitor_nominal_specify=off  v_capacitor_nominal_unit=V  v_capacitor_nominal_value=1  faulted_specify=off  faulted_priority=None  faulted=0  faulted_nominal_specify=off  faulted_nominal_unit=1  faulted_nominal_value=1  i_diode_specify=off  i_diode_priority=None  i_diode=0 A  i_diode_nominal_specify=off  i_diode_nominal_unit=A  i_diode_nominal_value=1  v_diode_specify=off  v_diode_priority=None  v_diode=0 V  v_diode_nominal_specify=off  v_diode_nominal_unit=V  v_diode_nominal_value=1  i_capacitor_specify=off  i_capacitor_priority=None  i_capacitor=0 A  i_capacitor_nominal_specify=off  i_capacitor_nominal_unit=A  i_capacitor_nominal_value=1  power_dissipated_specify=off  power_dissipated_priority=None  power_dissipated=0 W  power_dissipated_nominal_specify=off  power_dissipated_nominal_unit=W  power_dissipated_nominal_value=1  fidelity_level=ee.enum.diode.fidelity.includeChargeDyn  rec_loss_model=ee.enum.diode.reverseRecoveryModel.fixed  ErecVal=0 J  scaleWithIandV=true  ErecMat=zeros(2, 3) J  TjrecVec=[298.15, 398.15] K  IfrecVec=[.1, 1, 10] A  IrecVal=10 A  VrecVal=10 V  tFilter=1 / 1000 / 100 s  max_permissible_temperature=inf K  t_fail_on_temperature=1 s  thermal_network_parameterization=ee.enum.thermalNetworkTopology.junctionCase  Rth=[0, 10] K/W  Rth_Cauer=[1, 3, 10] K/W  Rth_Foster=[4, 6] K/W  thermal_mass_parameterization=ee.enum.thermalNetwork.timeconstant  thermal_mass=[0, 1] J/K  thermal_mass_Cauer=[.1, .3, 1] J/K  thermal_mass_Foster=[1.5, 3] J/K  thermal_time_constant=[0, 10] s  thermal_time_constant_Cauer=[1, 3, 10] s  thermal_time_constant_Foster=[6, 18] s  thermal_mass_initial_temperatures=[25, 25] degC  thermal_mass_initial_temperatures_Cauer=[25, 25, 25] degC  junction_thermal_mass=0.01 J/K  Tvec_initial_Foster=[25, 25, 25, 25] degC  no_thermal_network=0  junction_temperature_specify=off  junction_temperature_priority=None  junction_temperature=25 degC  junction_temperature_nominal_specify=off  junction_temperature_nominal_unit=degC  junction_temperature_nominal_value=1
  Resistor : fl_lib/Electrical/Electrical Elements/Resistor  R=33 Ohm  i_specify=off  i_priority=None  i=0 A  i_nominal_specify=off  i_nominal_unit=A  i_nominal_value=1  v_specify=off  v_priority=None  v=0 V  v_nominal_specify=off  v_nominal_unit=V  v_nominal_value=1
  Simulink-PS Converter : nesl_utility/Simulink-PS Converter  PhysicalDomain=network_engine_domain  SubClassName=ps_input  LeftPortType=input  RightPortType=output  PseudoPeriodic=off  Frequencies=[]  NoiseDistribution=none  NoiseParameters=[]  Unit=1  AffineConversion=off  FilteringAndDerivatives=provide  SimscapeFilterOrder=1  InputFilterTimeConstant=0.001  UdotUserProvided=0
  Switch : fl_lib/Electrical/Electrical Elements/Switch  R_closed=0.01 Ohm  G_open=1e-8 1/Ohm  Threshold=0.5  i_specify=off  i_priority=None  i=0 A  i_nominal_specify=off  i_nominal_unit=A  i_nominal_value=1  v_specify=off  v_priority=None  v=0 V  v_nominal_specify=off  v_nominal_unit=V  v_nominal_value=1
  +ve : PMIOPort  Side=Right
  -ve : PMIOPort  Port=2  Side=Right
  wires:
  Balance Command/1 -> Simulink-PS Converter/1
  connections:
  Diode/RConn1 -- Switch/LConn1
  Resistor/RConn1 -- Diode/LConn1
  Resistor/LConn1 -- +ve/RConn1
  -ve/RConn1 -- Switch/RConn2
  Simulink-PS Converter/RConn1 -- Switch/RConn1

== system Copy_of_BatteryPack/Subsystem3/Battery pack3/Subsystem6 ==
  Balance Command : Inport
  Diode : ee_lib/Semiconductors & Converters/Diode  ModelType=ee.enum.diode.modelType.pwl  TableType=ee.enum.diode.tableType.IfMat  IfMat=[.07, .12, .19, 1.75, 4.24, 7.32, 11.2; .16, .3, .72, 2.14, 5.02, 8.35, 13.12] A  VfMat=[.9, 1.15, 1.25, 1.5, 1.75, 2.17, 2.6, 2.85; .58, .68, .75, 1.1, 1.38, 1.77, 2.27, 2.7] V  TjVec=[25, 125] degC  VfVec=[.5, .7, .9, 1.3, 1.7, 2.1, 2.5] V  IfVec=[.1, .2, .5, 1, 2, 4, 7, 10] A  Vf=0.6 V  Ron=0.3 Ohm  Goff=1e-8 S  prmExp=ee.enum.diode.expParam.useTwo  I12=[.0137, .545] A  V12=[.6, .7] V  RS=0 Ohm  Tmeas=25 degC  IS=1e-12 A  ec=1  I1=0.0137 A  V1=0.6 V  N_series=1  N_parallel=1  ZenerEnable=false  Rz=0.3 Ohm  BV=inf V  C_param=ee.enum.diode.capParam.fixed  CJ=0 pF  CJ0=5 pF  Vvec=[.1, 10, 100] V  Cvec=[3.5, 1, .4] pF  VJ=1 V  Mgrad=0.5  FC=0.5  Q_param=ee.enum.diode.recoveryParam.off  iRM=-7.15 A  iF=4 A  didt=-750 A/us  trr_factor=3  trr=115 ns  Qrr=150 nA*s  Vr=-600 V  Ls=150 nH  Erec=0.03 J  TT=50 ns  tau=100 ns  T_param=ee.enum.diode.temperatureParam.off  Tdevice=25 degC  I1_T2=0.245 A  V1_T2=0.5 V  IS_T2=1.25e-7 A  Tmeas2=125 degC  XTI_param=ee.enum.diode.xtiParam.pn  XTI=3  EG_param=ee.enum.diode.egapParam.material_si  EG=1.11 eV  dBVdT=0 V/K  enable_faults=simscape.enum.onoff.off  fault_action=simscape.enum.assert.action.none  fault_types=ee.enum.diode.faults.open  tau_fault=1e-3 s  IfMat_faulted=[.07, .12, .19, 1.75, 4.24, 7.32, 11.2; .16, .3, .72, 2.14, 4.02, 6.35, 9.12] A  VfMat_faulted=[.9, 1.15, 1.25, 1.5, 1.75, 2.17, 2.6, 2.85; .58, .68, .75, 1.1, 1.38, 1.77, 2.27, 2.7] V  VfVec_faulted=[.5, .7, .9, 1.3, 1.7, 2.1, 2.5] V  IfVec_faulted=[.1, .2, .5, 1, 2, 4, 7, 10] A  Ropen_faulted=1000 Ohm  Gshort_faulted=1000 1/Ohm  Vf_faulted=0.6 V  Ron_faulted=0.3 Ohm  Goff_faulted=1e-8 S  I12_faulted=[.0137, .545] A  V12_faulted=[.6, .7] V  IS_faulted=1e-12 A  ec_faulted=1  I1_faulted=0.0137 A  V1_faulted=0.6 V  RS_faulted=0 Ohm  Rz_faulted=0.3 Ohm  BV_faulted=inf V  Cscale_faulted=100  fault_trigger=ee.enum.faults.faultTrigger.temporal  t_fault=inf s  max_permissible_voltage=inf V  n_fail_on_voltage=1  max_permissible_current=inf A  t_fail_on_current=1 s  max_permissible_dVdt=inf V/s  enable_fault_input=simscape.enum.onoff.off  i_specify=off  i_priority=None  i=0 A  i_nominal_specify=off  i_nominal_unit=A  i_nominal_value=1  v_specify=off  v_priority=None  v=0 V  v_nominal_specify=off  v_nominal_unit=V  v_nominal_value=1  v_capacitor_specify=off  v_capacitor_priority=None  v_capacitor=0 V  v_capacitor_nominal_specify=off  v_capacitor_nominal_unit=V  v_capacitor_nominal_value=1  faulted_specify=off  faulted_priority=None  faulted=0  faulted_nominal_specify=off  faulted_nominal_unit=1  faulted_nominal_value=1  i_diode_specify=off  i_diode_priority=None  i_diode=0 A  i_diode_nominal_specify=off  i_diode_nominal_unit=A  i_diode_nominal_value=1  v_diode_specify=off  v_diode_priority=None  v_diode=0 V  v_diode_nominal_specify=off  v_diode_nominal_unit=V  v_diode_nominal_value=1  i_capacitor_specify=off  i_capacitor_priority=None  i_capacitor=0 A  i_capacitor_nominal_specify=off  i_capacitor_nominal_unit=A  i_capacitor_nominal_value=1  power_dissipated_specify=off  power_dissipated_priority=None  power_dissipated=0 W  power_dissipated_nominal_specify=off  power_dissipated_nominal_unit=W  power_dissipated_nominal_value=1  fidelity_level=ee.enum.diode.fidelity.includeChargeDyn  rec_loss_model=ee.enum.diode.reverseRecoveryModel.fixed  ErecVal=0 J  scaleWithIandV=true  ErecMat=zeros(2, 3) J  TjrecVec=[298.15, 398.15] K  IfrecVec=[.1, 1, 10] A  IrecVal=10 A  VrecVal=10 V  tFilter=1 / 1000 / 100 s  max_permissible_temperature=inf K  t_fail_on_temperature=1 s  thermal_network_parameterization=ee.enum.thermalNetworkTopology.junctionCase  Rth=[0, 10] K/W  Rth_Cauer=[1, 3, 10] K/W  Rth_Foster=[4, 6] K/W  thermal_mass_parameterization=ee.enum.thermalNetwork.timeconstant  thermal_mass=[0, 1] J/K  thermal_mass_Cauer=[.1, .3, 1] J/K  thermal_mass_Foster=[1.5, 3] J/K  thermal_time_constant=[0, 10] s  thermal_time_constant_Cauer=[1, 3, 10] s  thermal_time_constant_Foster=[6, 18] s  thermal_mass_initial_temperatures=[25, 25] degC  thermal_mass_initial_temperatures_Cauer=[25, 25, 25] degC  junction_thermal_mass=0.01 J/K  Tvec_initial_Foster=[25, 25, 25, 25] degC  no_thermal_network=0  junction_temperature_specify=off  junction_temperature_priority=None  junction_temperature=25 degC  junction_temperature_nominal_specify=off  junction_temperature_nominal_unit=degC  junction_temperature_nominal_value=1
  Resistor : fl_lib/Electrical/Electrical Elements/Resistor  R=33 Ohm  i_specify=off  i_priority=None  i=0 A  i_nominal_specify=off  i_nominal_unit=A  i_nominal_value=1  v_specify=off  v_priority=None  v=0 V  v_nominal_specify=off  v_nominal_unit=V  v_nominal_value=1
  Simulink-PS Converter : nesl_utility/Simulink-PS Converter  PhysicalDomain=network_engine_domain  SubClassName=ps_input  LeftPortType=input  RightPortType=output  PseudoPeriodic=off  Frequencies=[]  NoiseDistribution=none  NoiseParameters=[]  Unit=1  AffineConversion=off  FilteringAndDerivatives=provide  SimscapeFilterOrder=1  InputFilterTimeConstant=0.001  UdotUserProvided=0
  Switch : fl_lib/Electrical/Electrical Elements/Switch  R_closed=0.01 Ohm  G_open=1e-8 1/Ohm  Threshold=0.5  i_specify=off  i_priority=None  i=0 A  i_nominal_specify=off  i_nominal_unit=A  i_nominal_value=1  v_specify=off  v_priority=None  v=0 V  v_nominal_specify=off  v_nominal_unit=V  v_nominal_value=1
  +ve : PMIOPort  Side=Right
  -ve : PMIOPort  Port=2  Side=Right
  wires:
  Balance Command/1 -> Simulink-PS Converter/1
  connections:
  Diode/RConn1 -- Switch/LConn1
  Resistor/RConn1 -- Diode/LConn1
  Resistor/LConn1 -- +ve/RConn1
  -ve/RConn1 -- Switch/RConn2
  Simulink-PS Converter/RConn1 -- Switch/RConn1
